simulink model "four_RWs_four"  (R2024a)
settings: Solver=VariableStepAuto  StartTime=0.0  StopTime=180  RelTol=1e-3
undefined symbols (not defined in the file): initialRate
libraries: simulink_extras x3, matrix_library x1
settings Model: Creator=Dsipt  LastModifiedBy=Dsipt

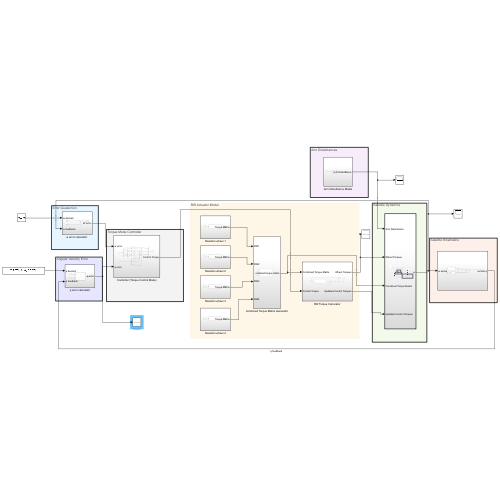
[thumbnail: Simulink's stored preview of the top-level diagram]
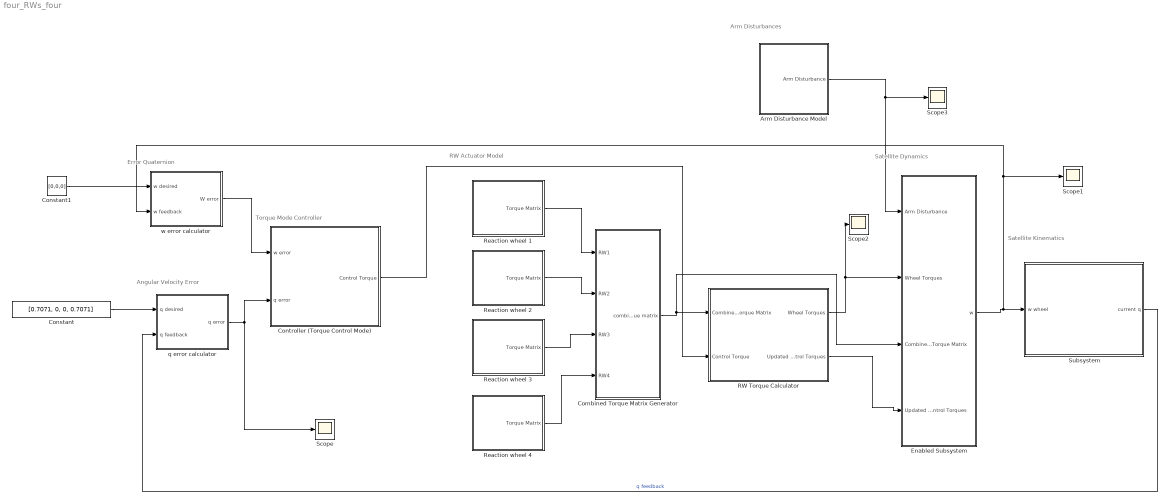
== system four_RWs_four ==
  note: Satellite Kinematics
  note: Arm Disturbances
  note: Satellite Dynamics
  note: RW Actuator Model
  note: Angular Velocity Error
  note: Error Quaternion
  note: Torque Mode Controller
  Arm Disturbance Model : Subsystem
  Combined Torque Matrix Generator : Subsystem
  Constant : Constant  Value=[0.7071, 0, 0, 0.7071]
  Constant1 : Constant  Value=[0,0,0]
  Controller (Torque Control Mode) : Subsystem
  Enabled Subsystem : Subsystem  TreatAsAtomicUnit=on
  RW Torque Calculator : Subsystem
  Reaction wheel 1 : Subsystem
  Reaction wheel 2 : Subsystem
  Reaction wheel 3 : Subsystem
  Reaction wheel 4 : Subsystem
  Scope{,1..3} (4 alike) : Scope
  Subsystem : Subsystem
  q error calculator : Subsystem
  "w error calculator " : Subsystem
  wires:
  "w error calculator "/1(W error) -> Controller (Torque Control Mode)/1(w error)
  q error calculator/1(q error) -> Scope/1, Controller (Torque Control Mode)/2(q error)
  Subsystem/1(current q) -> q error calculator/2(q feedback)  "q feedback"
  Reaction wheel 1/1(Torque Matrix) -> Combined Torque Matrix Generator/1(RW1)
  Reaction wheel 2/1(Torque Matrix) -> Combined Torque Matrix Generator/2(RW2)
  Reaction wheel 4/1(Torque Matrix) -> Combined Torque Matrix Generator/4(RW4)
  Reaction wheel 3/1(Torque Matrix) -> Combined Torque Matrix Generator/3(RW3)
  Controller (Torque Control Mode)/1(Control Torque) -> RW Torque Calculator/2(Control Torque)
  RW Torque Calculator/1(Wheel Torques) -> Enabled Subsystem/2(Wheel Torques), Scope2/1
  RW Torque Calculator/2(Updated Control Torques) -> Enabled Subsystem/4(Updated Control Torques)
  Combined Torque Matrix Generator/1(combind torque matrix) -> Enabled Subsystem/3(Combined Torque Matrix), RW Torque Calculator/1(Combined Torque Matrix)
  Constant/1 -> q error calculator/1(q desired)
  Constant1/1 -> "w error calculator "/1(w desired)
  Enabled Subsystem/1(w) -> Scope1/1, "w error calculator "/2(w feedback), Subsystem/1(w wheel)
  Arm Disturbance Model/1(Arm Disturbance) -> Scope3/1, Enabled Subsystem/1(Arm Disturbance)

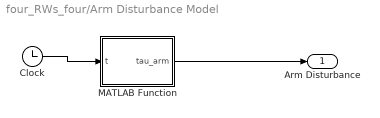
== system four_RWs_four/Arm Disturbance Model ==
  Clock : Clock
  MATLAB Function : MATLAB Function  TreatAsAtomicUnit=on
  Arm Disturbance : Outport
  wires:
  Clock/1 -> MATLAB Function/1(t)
  MATLAB Function/1(tau_arm) -> Arm Disturbance/1

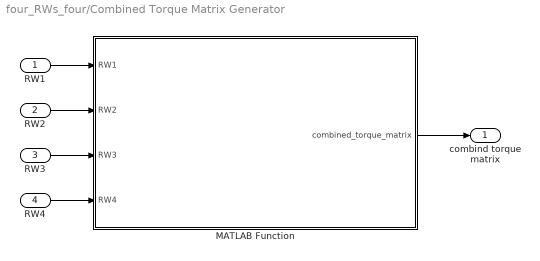
== system four_RWs_four/Combined Torque Matrix Generator ==
  RW1 : Inport
  RW2 : Inport  Port=2
  RW3 : Inport  Port=3
  RW4 : Inport  Port=4
  MATLAB Function : MATLAB Function  TreatAsAtomicUnit=on
  combind torque matrix : Outport
  wires:
  RW1/1 -> MATLAB Function/1(RW1)
  RW2/1 -> MATLAB Function/2(RW2)
  RW3/1 -> MATLAB Function/3(RW3)
  RW4/1 -> MATLAB Function/4(RW4)
  MATLAB Function/1(combined_torque_matrix) -> combind torque matrix/1

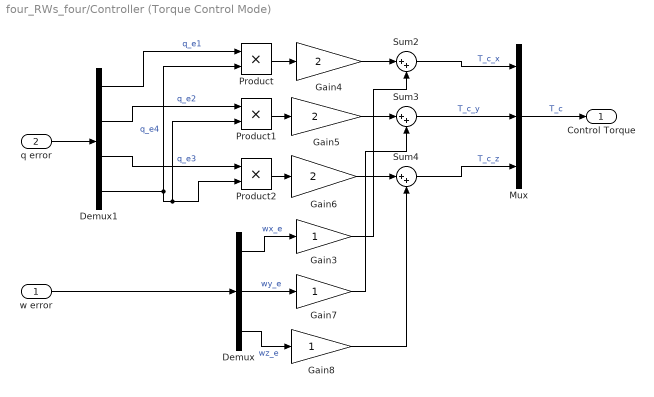
== system four_RWs_four/Controller (Torque Control Mode) ==
  w error : Inport
  q error : Inport  Port=2
  Demux : Demux  Outputs=3
  Demux1 : Demux
  Gain3 : Gain
  Gain4 : Gain  Gain=2
  Gain5 : Gain  Gain=2
  Gain6 : Gain  Gain=2
  Gain7 : Gain
  Gain8 : Gain
  Mux : Mux  Inputs=3
  Product : Product
  Product1 : Product
  Product2 : Product
  Sum2 : Sum  Inputs=|++
  Sum3 : Sum  Inputs=|++
  Sum4 : Sum  Inputs=|++
  Control Torque : Outport
  wires:
  Gain5/1 -> Sum3/1
  Gain3/1 -> Sum2/2
  Demux/2 -> Gain7/1  "wy_e"
  Gain6/1 -> Sum4/1
  Demux/1 -> Gain3/1  "wx_e"
  Gain7/1 -> Sum3/2
  Mux/1 -> Control Torque/1  "T_c"
  Sum4/1 -> Mux/3  "T_c_z"
  Sum3/1 -> Mux/2  "T_c_y"
  Sum2/1 -> Mux/1  "T_c_x"
  Product1/1 -> Gain5/1
  Product2/1 -> Gain6/1
  Demux/3 -> Gain8/1  "wz_e"
  Product/1 -> Gain4/1
  Demux1/1 -> Product/1  "q_e1"
  Gain4/1 -> Sum2/1
  Demux1/2 -> Product1/1  "q_e2"
  Demux1/4 -> Product1/2, Product2/2, Product/2  "q_e4"
  Demux1/3 -> Product2/1  "q_e3"
  w error/1 -> Demux/1
  Gain8/1 -> Sum4/2
  q error/1 -> Demux1/1

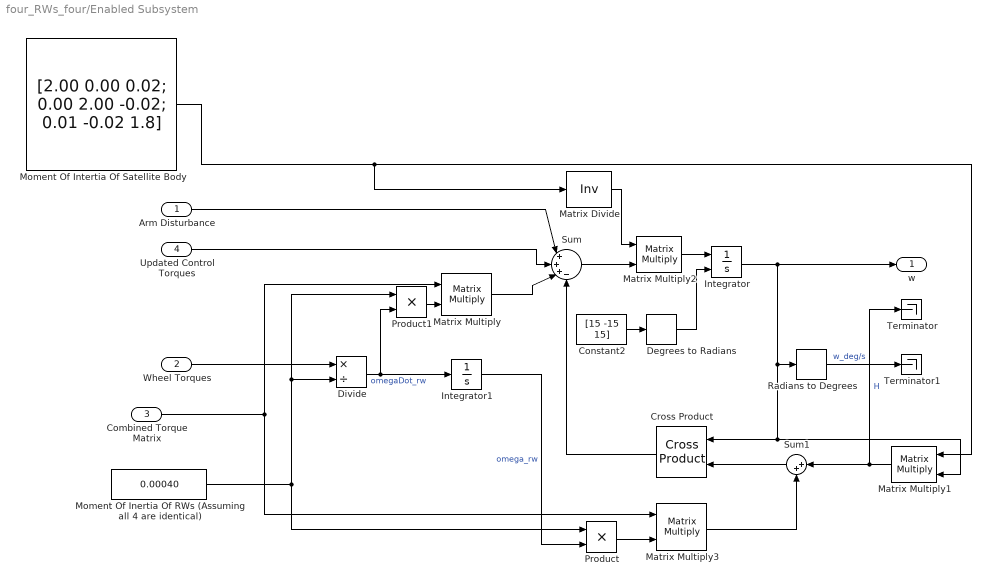
== system four_RWs_four/Enabled Subsystem ==
  Arm Disturbance : Inport
  Wheel Torques : Inport  Port=2
  Combined Torque Matrix : Inport  Port=3
  Updated Control Torques : Inport  Port=4
  Constant2 : Constant  Value=[15 -15 15]
  Cross Product : matrix_library/Cross Product
  Degrees to Radians : simulink_extras/Transformations/Degrees to Radians
  Divide : Product  Inputs=*/
  Integrator : Integrator  InitialConditionSource=external  InitialCondition=initialRate
  Integrator1 : Integrator  InitialCondition=zeros(4,1)
  Matrix Divide : Product  Inputs=/  Multiplication=Matrix(*)
  Matrix Multiply{,1..3} (4 alike) : Product  Multiplication=Matrix(*)
  Moment Of Inertia Of RWs (Assuming all 4 are identical) : Constant  Value=0.00040
  Moment Of Intertia Of Satellite Body : Constant  Value=|
      | [2.00 0.00 0.02;
      |                 0.00 2.00 -0.02;
      |                 0.01 -0.02 1.8]
  Product : Product
  Product1 : Product
  Radians to Degrees : simulink_extras/Transformations/Radians to Degrees
  Sum : Sum  Inputs=|+++-
  Sum1 : Sum  Inputs=|++
  Terminator : Terminator
  Terminator1 : Terminator
  w : Outport
  wires:
  Combined Torque Matrix/1 -> Matrix Multiply3/1, Matrix Multiply/1
  Arm Disturbance/1 -> Sum/1
  Product1/1 -> Matrix Multiply/2
  Sum1/1 -> Cross Product/2
  Sum/1 -> Matrix Multiply2/2
  Matrix Multiply1/1 -> Terminator/1, Sum1/1  "H"
  Moment Of Inertia Of RWs (Assuming all 4 are identical)/1 -> Product1/1, Divide/2, Product/1
  Degrees to Radians/1 -> Integrator/2
  Matrix Multiply2/1 -> Integrator/1
  Divide/1 -> Integrator1/1, Product1/2  "omegaDot_rw"
  Integrator/1 -> w/1, Matrix Multiply1/2, Cross Product/1, Radians to Degrees/1
  Moment Of Intertia Of Satellite Body/1 -> Matrix Divide/1, Matrix Multiply1/1
  Radians to Degrees/1 -> Terminator1/1  "w_deg/s"
  Constant2/1 -> Degrees to Radians/1
  Matrix Multiply3/1 -> Sum1/2
  Product/1 -> Matrix Multiply3/2
  Matrix Divide/1 -> Matrix Multiply2/1
  Cross Product/1 -> Sum/4
  Updated Control Torques/1 -> Sum/2
  Wheel Torques/1 -> Divide/1
  Matrix Multiply/1 -> Sum/3
  Integrator1/1 -> Product/2  "omega_rw"

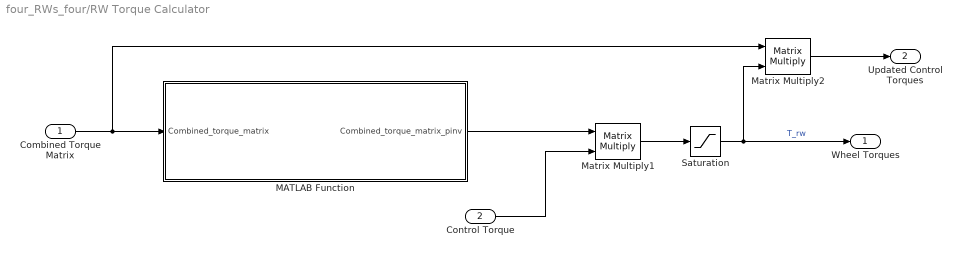
== system four_RWs_four/RW Torque Calculator ==
  Combined Torque Matrix : Inport
  Control Torque : Inport  Port=2
  MATLAB Function : MATLAB Function  TreatAsAtomicUnit=on
  Matrix Multiply1 : Product  Multiplication=Matrix(*)
  Matrix Multiply2 : Product  Multiplication=Matrix(*)
  Saturation : Saturate  UpperLimit=0.02  LowerLimit=-0.02
  Wheel Torques : Outport
  Updated Control Torques : Outport  Port=2
  wires:
  Combined Torque Matrix/1 -> Matrix Multiply2/1, MATLAB Function/1(Combined_torque_matrix)
  MATLAB Function/1(Combined_torque_matrix_pinv) -> Matrix Multiply1/1
  Control Torque/1 -> Matrix Multiply1/2
  Matrix Multiply1/1 -> Saturation/1
  Saturation/1 -> Wheel Torques/1, Matrix Multiply2/2  "T_rw"
  Matrix Multiply2/1 -> Updated Control Torques/1

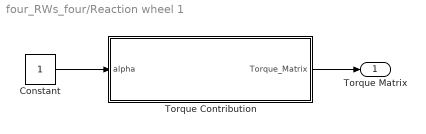
== system four_RWs_four/Reaction wheel 1 ==
  Constant : Constant
  Torque Contribution : MATLAB Function  TreatAsAtomicUnit=on
  Torque Matrix : Outport
  wires:
  Constant/1 -> Torque Contribution/1(alpha)
  Torque Contribution/1(Torque_Matrix) -> Torque Matrix/1

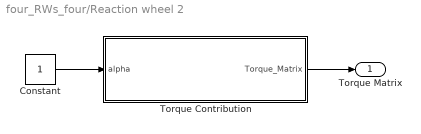
== system four_RWs_four/Reaction wheel 2 ==
  Constant : Constant
  Torque Contribution : MATLAB Function  TreatAsAtomicUnit=on
  Torque Matrix : Outport
  wires:
  Torque Contribution/1(Torque_Matrix) -> Torque Matrix/1
  Constant/1 -> Torque Contribution/1(alpha)

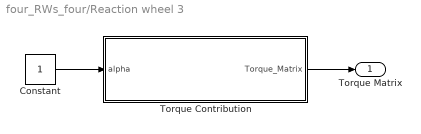
== system four_RWs_four/Reaction wheel 3 ==
  Constant : Constant
  Torque Contribution : MATLAB Function  TreatAsAtomicUnit=on
  Torque Matrix : Outport
  wires:
  Torque Contribution/1(Torque_Matrix) -> Torque Matrix/1
  Constant/1 -> Torque Contribution/1(alpha)

== system four_RWs_four/Reaction wheel 4 ==
  Constant : Constant
  Torque Contribution : MATLAB Function  TreatAsAtomicUnit=on
  Torque Matrix : Outport
  wires:
  Torque Contribution/1(Torque_Matrix) -> Torque Matrix/1
  Constant/1 -> Torque Contribution/1(alpha)

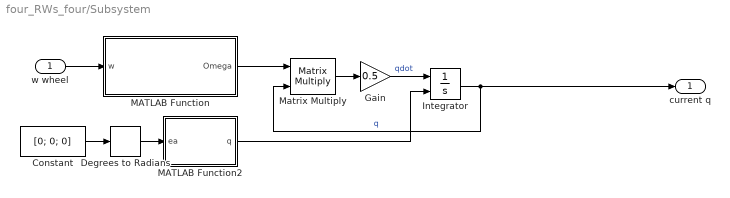
== system four_RWs_four/Subsystem ==
  w wheel : Inport
  Constant : Constant  Value=[0; 0; 0]
  Degrees to Radians : simulink_extras/Transformations/Degrees to Radians
  Gain : Gain  Gain=0.5
  Integrator : Integrator  InitialConditionSource=external  InitialCondition=[1; 0; 0; 0]
  MATLAB Function : MATLAB Function  TreatAsAtomicUnit=on
  MATLAB Function2 : MATLAB Function  TreatAsAtomicUnit=on
  Matrix Multiply : Product  Multiplication=Matrix(*)
  current q : Outport
  wires:
  Degrees to Radians/1 -> MATLAB Function2/1(ea)
  MATLAB Function2/1(q) -> Integrator/2
  Constant/1 -> Degrees to Radians/1
  Gain/1 -> Integrator/1  "qdot"
  MATLAB Function/1(Omega) -> Matrix Multiply/1
  w wheel/1 -> MATLAB Function/1(w)
  Integrator/1 -> current q/1, Matrix Multiply/2  "q"
  Matrix Multiply/1 -> Gain/1

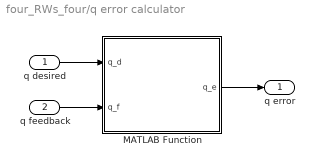
== system four_RWs_four/q error calculator ==
  q desired : Inport
  q feedback : Inport  Port=2
  MATLAB Function : MATLAB Function  TreatAsAtomicUnit=on
  q error : Outport
  wires:
  q feedback/1 -> MATLAB Function/2(q_f)
  MATLAB Function/1(q_e) -> q error/1
  q desired/1 -> MATLAB Function/1(q_d)

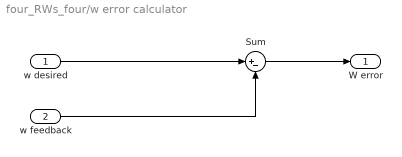
== system four_RWs_four/w error calculator  ==
  w desired : Inport
  w feedback : Inport  Port=2
  Sum : Sum  Inputs=|+-
  W error : Outport
  wires:
  w desired/1 -> Sum/1
  Sum/1 -> W error/1
  w feedback/1 -> Sum/2

== matlab function four_RWs_four/q error calculator/MATLAB Function ==
  data: q_d input; q_e output; q_f input
%Made By DRS46 
%Function that inputs desired quaternion (from wanted attitude) and
%calculates the error based on the current quaternion of the SACS 

%All in standard form [x, y, z, w] where w is the scalar component

function q_e = q_error_calculator(q_d,q_f)

%Extracts x,y,z and scalar components
x = q_d(1); 
y = q_d(2);
z = q_d(3); 
scalar = q_d(4);


%Calculates the conjugate quaternion of q feedback 
q_c = [-q_f(1); -q_f(2); -q_f(3); q_f(4)];

%Builds the 4x4 multiplication matrix for q desired
Q_d = zeros(4,4);
Q_d(1,:) = [ scalar,  z, -y,  x];
Q_d(2,:) = [-z,  scalar,  x,  y];
Q_d(3,:) = [ y, -x,  scalar,  z];
Q_d(4,:) = [-x, -y, -z,  scalar];

%Computes the error quaternion with a 0.5 Scalar component to allow for
%simulation efficiency 
q_e = 0.5 * Q_d * q_c;
end

== matlab function four_RWs_four/Subsystem/MATLAB Function ==
  data: w input; Omega output
function Omega = fcn(w)

wx = w(1,1);
wy = w(2,1);
wz = w(3,1);

Omega = [0,  wz, -wy,  wx;
       -wz,   0,  wx, wy;
        wy, -wx,   0,  wz;
       -wx, -wy, -wz,  0];

== matlab function four_RWs_four/Subsystem/MATLAB Function2 ==
  data: ea input; q output
function q = fcn(ea)

phi = ea(1,1);
theta = ea(2,1);
psi = ea(3,1);

q1 =  sin(psi/2)*sin(theta/2)*sin(phi/2) + cos(psi/2)*cos(theta/2)*cos(phi/2);
q2 = -sin(psi/2)*sin(theta/2)*cos(phi/2) + cos(psi/2)*cos(theta/2)*sin(phi/2);
q3 =  sin(psi/2)*cos(theta/2)*sin(phi/2) + cos(psi/2)*sin(theta/2)*cos(phi/2);
q4 =  sin(psi/2)*cos(theta/2)*cos(phi/2) - cos(psi/2)*sin(theta/2)*sin(phi/2);

q = [q1; q2; q3; q4];

== matlab function four_RWs_four/Reaction wheel 1/Torque Contribution ==
  data: alpha input; Torque_Matrix output
function Torque_Matrix= config_RW_Matrix(alpha)

Torque_Matrix = [cos(alpha);0;sin(alpha)];

end

== matlab function four_RWs_four/Reaction wheel 2/Torque Contribution ==
  data: alpha input; Torque_Matrix output
function Torque_Matrix= config_RW_Matrix(alpha)

Torque_Matrix = [0;cos(alpha);sin(alpha)];

end

== matlab function four_RWs_four/Reaction wheel 3/Torque Contribution ==
  data: alpha input; Torque_Matrix output
function Torque_Matrix= config_RW_Matrix(alpha)

% Torque_Matrix = [-cos(alpha);0;sin(alpha)];
 Torque_Matrix = [0;0;0];
end

== matlab function four_RWs_four/Arm Disturbance Model/MATLAB Function ==
  data: t input; tau_arm output
function tau_arm = arm_disturbance_torque(t)
%PLAN FOR THE MISSION EXAMPLE
% t = 0–10s: idle
% t = 10–30s: Arm Start Moving (medium to Low torque)
% t = 30–50s: fast Moving (high torque As Arm move)
% t = 50–70s: hold (small Torque as Repair takes place)
% t = 70–100s: retract (moderate torque As arm is retracted and repair is completed)
tau_arm = zeros(3,1); %Creates 3-axes out
%Mission parameter from 0 to 10s
if t >= 10 && t < 30
    tau_arm(1) = 0.02 * sin(0.5 * t); % Nm in X
    tau_arm(2) = 0.015 * sin(0.6 * t); % Nm in Y
    tau_arm(3) = 0.01 * sin(0.4 * t);  % Nm in Z
%Mission parameter from 30 to 50s
elseif t >= 30 && t < 50
    tau_arm(1) = 0.05 * sin(0.7 * t);
    tau_arm(2) = 0.04 * sin(0.8 * t + 0.5);
    tau_arm(3) = 0.03 * sin(0.6 * t + 1);
%Mission parameter from 50 to 70s
elseif t >= 50 && t < 70
    tau_arm(1) = 0.005 * sin(0.3 * t);
    tau_arm(2) = 0.005 * sin(0.3 * t);
    tau_arm(3) = 0.005 * sin(0.3 * t);
%Mission parameter from 70 to 100s
elseif t >= 70 && t <= 100
    tau_arm(1) = 0.02 * sin(0.5 * t + 1);
    tau_arm(2) = 0.015 * sin(0.6 * t);
    tau_arm(3) = 0.01 * sin(0.4 * t + 0.5);
end
end

== matlab function four_RWs_four/Reaction wheel 4/Torque Contribution ==
  data: alpha input; Torque_Matrix output
function Torque_Matrix= config_RW_Matrix(alpha)

Torque_Matrix = [0;-cos(alpha);sin(alpha)];

end

== matlab function four_RWs_four/RW Torque Calculator/MATLAB Function ==
  data: Combined_torque_matrix input; Combined_torque_matrix_pinv output
function Combined_torque_matrix_pinv = torque_pinv_matrix(Combined_torque_matrix)
%Creates a pseudo inverse of the Non-square Matrix which will then be used
%to create map the opposite of the body torques (i.e the reaction wheel torque)
Combined_torque_matrix_pinv = pinv(Combined_torque_matrix);

== matlab function four_RWs_four/Combined Torque Matrix Generator/MATLAB Function ==
  data: RW1 input; combined_torque_matrix output; RW2 input; RW3 input; RW4 input
function combined_torque_matrix = fcn(RW1,RW2,RW3,RW4)
    
combined_torque_matrix = [RW1,RW2,RW3,RW4];
